simulink model "ukol1"  (R2024b)
settings: Solver=VariableStepAuto  StartTime=0.0  StopTime=40000  RelTol=1e-3
settings Model: Creator=jirka  LastModifiedBy=jirka

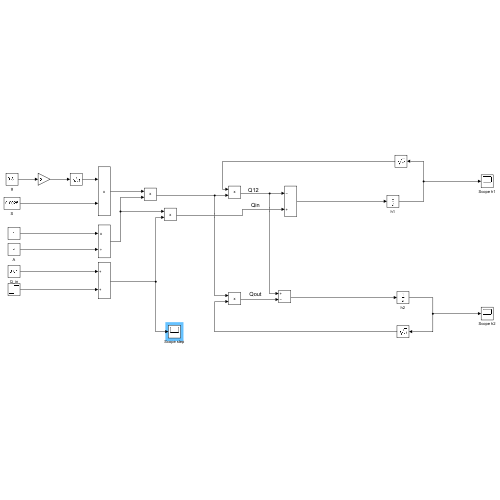
[thumbnail: Simulink's stored preview of the top-level diagram]
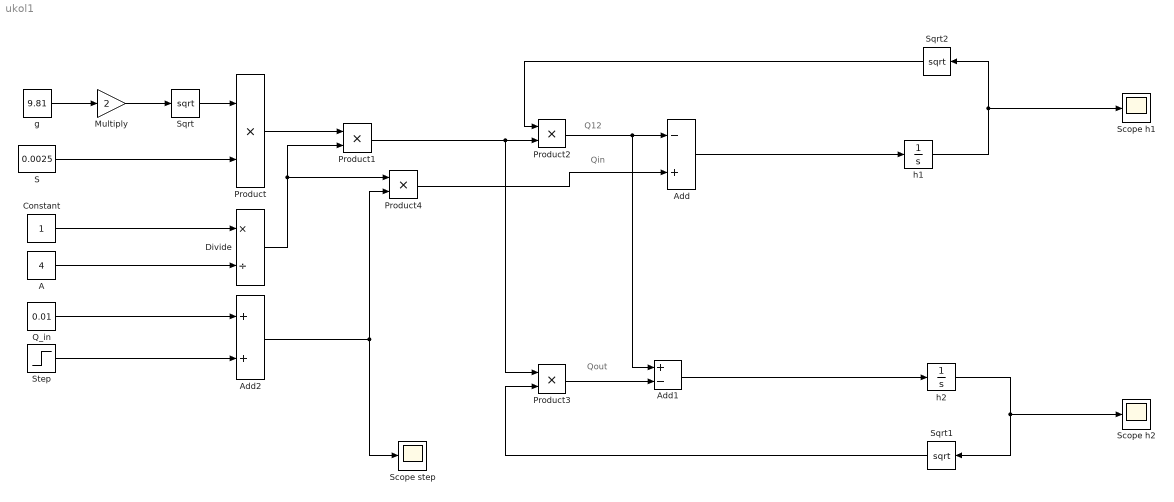
== system ukol1 ==
  note: Qin
  note: Qout
  note: Q12
  A : Constant  Value=4
  Add : Sum  Inputs=-+
  Add1 : Sum  Inputs=+-
  Add2 : Sum
  Constant : Constant
  Divide : Product  Inputs=*/
  Multiply : Gain  Gain=2
  Product{,1..4} (5 alike) : Product
  Q_in : Constant  Value=0.01
  S : Constant  Value=0.0025
  Scope h1 : Scope
  Scope h2 : Scope
  Scope step : Scope
  Sqrt : Sqrt
  Sqrt1 : Sqrt
  Sqrt2 : Sqrt
  Step : Step  Time=20000  After=0.001  SampleTime=0
  g : Constant  Value=9.81
  h1 : Integrator  InitialCondition=0.82
  h2 : Integrator  InitialCondition=0.82
  wires:
  g/1 -> Multiply/1
  Multiply/1 -> Sqrt/1
  Sqrt/1 -> Product/1
  S/1 -> Product/2
  Constant/1 -> Divide/1
  A/1 -> Divide/2
  Product/1 -> Product1/1
  Divide/1 -> Product4/1, Product1/2
  h2/1 -> Scope h2/1, Sqrt1/1
  h1/1 -> Scope h1/1, Sqrt2/1
  Product2/1 -> Add/1, Add1/1
  Sqrt2/1 -> Product2/1
  Product1/1 -> Product3/1, Product2/2
  Sqrt1/1 -> Product3/2
  Product3/1 -> Add1/2
  Step/1 -> Add2/2
  Q_in/1 -> Add2/1
  Add2/1 -> Product4/2, Scope step/1
  Add/1 -> h1/1
  Add1/1 -> h2/1
  Product4/1 -> Add/2
